simulink model "Follower_V2V_SelfSteer"  (R2014b)
settings: Solver=ode3  StartTime=0.0  StopTime=10.0  FixedStep=sampleTimes.main  RelTol=1e-3
model workspace (MAT data in the model file):
  spacing = 0
  vehicle = 0
undefined symbols (not defined in the file or in its folder): delays, sampleTimes
libraries: simulink x12
settings Model: ParameterArgumentNames=vehicle,spacing  Creator=uos  LastModifiedBy=uos

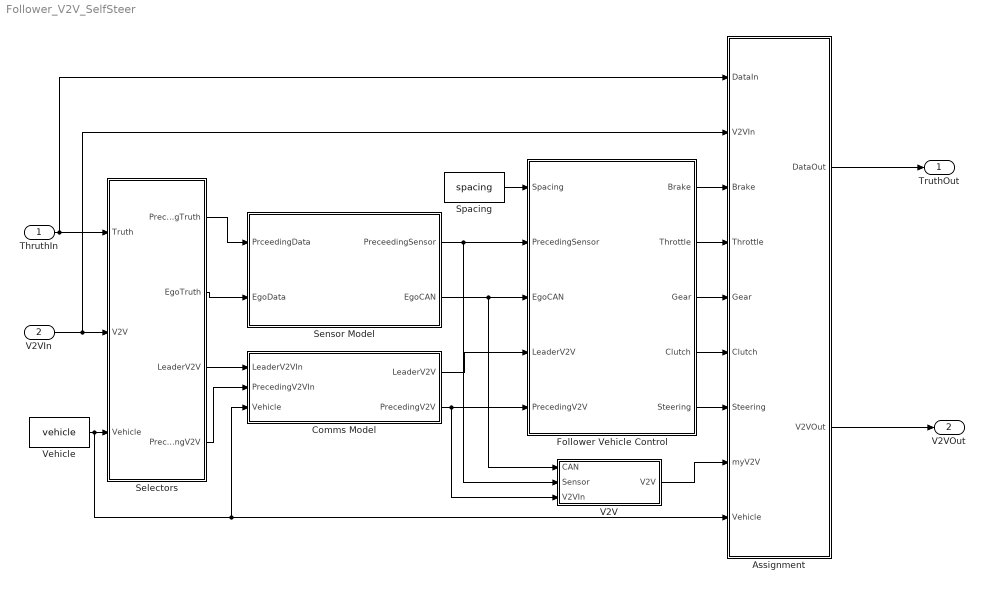
== system Follower_V2V_SelfSteer ==
  ThruthIn : Inport  OutDataTypeStr=Bus: VehicleBus  PortDimensions=10  BusOutputAsStruct=on
  V2VIn : Inport  Port=2  OutDataTypeStr=Bus: V2VBus  PortDimensions=10  SampleTime=0  BusOutputAsStruct=on
  Assignment : Subsystem
  Comms Model : Subsystem
  Follower Vehicle Control : Subsystem
  Selectors : Subsystem
  Sensor Model : Subsystem
  Spacing : Constant  Value=spacing
  V2V : Subsystem
  Vehicle : Constant  Value=vehicle
  TruthOut : Outport  OutDataTypeStr=Bus: VehicleBus  PortDimensions=10  BusOutputAsStruct=on
  V2VOut : Outport  Port=2  OutDataTypeStr=Bus: V2VBus  PortDimensions=10  BusOutputAsStruct=on
  wires:
  ThruthIn/1 -> Selectors/1(Truth), Assignment/1(DataIn)
  Assignment/1(DataOut) -> TruthOut/1
  Sensor Model/2(EgoCAN) -> V2V/1(CAN), Follower Vehicle Control/3(EgoCAN)
  Spacing/1 -> Follower Vehicle Control/1(Spacing)
  Sensor Model/1(PreceedingSensor) -> V2V/2(Sensor), Follower Vehicle Control/2(PrecedingSensor)
  Selectors/1(PrecedingTruth) -> Sensor Model/1(PrceedingData)
  Selectors/2(EgoTruth) -> Sensor Model/2(EgoData)
  Vehicle/1 -> Assignment/9(Vehicle), Comms Model/3(Vehicle), Selectors/3(Vehicle)
  Follower Vehicle Control/1(Brake) -> Assignment/3(Brake)
  Follower Vehicle Control/2(Throttle) -> Assignment/4(Throttle)
  Follower Vehicle Control/3(Gear) -> Assignment/5(Gear)
  Follower Vehicle Control/4(Clutch) -> Assignment/6(Clutch)
  Follower Vehicle Control/5(Steering) -> Assignment/7(Steering)
  Selectors/3(LeaderV2V) -> Comms Model/1(LeaderV2VIn)
  Selectors/4(PrecedingV2V) -> Comms Model/2(PrecedingV2VIn)
  Comms Model/1(LeaderV2V) -> Follower Vehicle Control/4(LeaderV2V)
  Comms Model/2(PrecedingV2V) -> V2V/3(V2VIn), Follower Vehicle Control/5(PrecedingV2V)
  V2V/1(V2V) -> Assignment/8(myV2V)
  V2VIn/1 -> Assignment/2(V2VIn), Selectors/2(V2V)
  Assignment/2(V2VOut) -> V2VOut/1

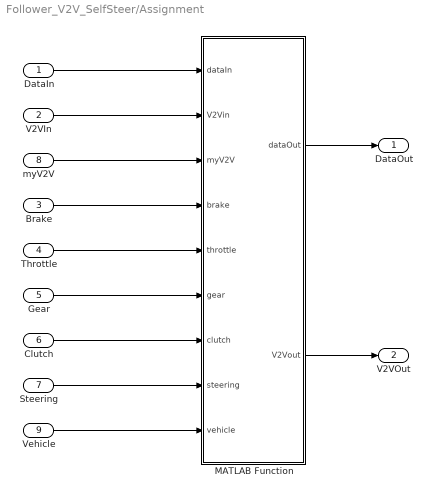
== system Follower_V2V_SelfSteer/Assignment ==
  DataIn : Inport
  V2VIn : Inport  Port=2
  Brake : Inport  Port=3
  Throttle : Inport  Port=4
  Gear : Inport  Port=5
  Clutch : Inport  Port=6
  Steering : Inport  Port=7
  myV2V : Inport  Port=8
  Vehicle : Inport  Port=9
  MATLAB Function : MATLAB Function  TreatAsAtomicUnit=on
  DataOut : Outport
  V2VOut : Outport  Port=2
  wires:
  Vehicle/1 -> MATLAB Function/9(vehicle)
  DataIn/1 -> MATLAB Function/1(dataIn)
  Brake/1 -> MATLAB Function/4(brake)
  MATLAB Function/1(dataOut) -> DataOut/1
  Throttle/1 -> MATLAB Function/5(throttle)
  Gear/1 -> MATLAB Function/6(gear)
  Clutch/1 -> MATLAB Function/7(clutch)
  Steering/1 -> MATLAB Function/8(steering)
  V2VIn/1 -> MATLAB Function/2(V2Vin)
  myV2V/1 -> MATLAB Function/3(myV2V)
  MATLAB Function/2(V2Vout) -> V2VOut/1

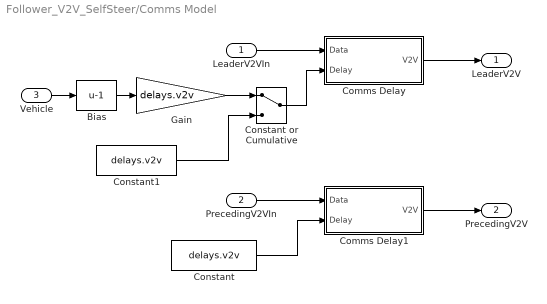
== system Follower_V2V_SelfSteer/Comms Model ==
  LeaderV2VIn : Inport
  PrecedingV2VIn : Inport  Port=2
  Vehicle : Inport  Port=3
  Bias : Bias  Bias=-1
  Comms Delay : Subsystem
  Comms Delay1 : Subsystem
  Constant : Constant  Value=delays.v2v
  Constant or Cumulative : ManualSwitch
  Constant1 : Constant  Value=delays.v2v
  Gain : Gain  Gain=delays.v2v
  LeaderV2V : Outport
  PrecedingV2V : Outport  Port=2
  wires:
  LeaderV2VIn/1 -> Comms Delay/1(Data)
  Comms Delay/1(V2V) -> LeaderV2V/1
  PrecedingV2VIn/1 -> Comms Delay1/1(Data)
  Comms Delay1/1(V2V) -> PrecedingV2V/1
  Constant/1 -> Comms Delay1/2(Delay)
  Constant or Cumulative/1 -> Comms Delay/2(Delay)
  Constant1/1 -> Constant or Cumulative/2
  Vehicle/1 -> Bias/1
  Bias/1 -> Gain/1
  Gain/1 -> Constant or Cumulative/1

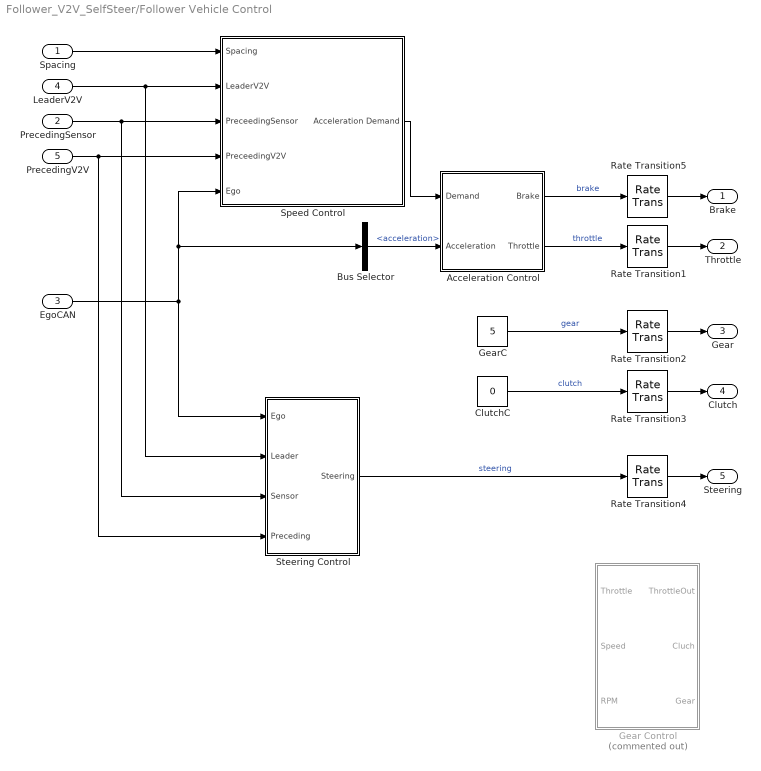
== system Follower_V2V_SelfSteer/Follower Vehicle Control ==
  Spacing : Inport
  PrecedingSensor : Inport  Port=2
  EgoCAN : Inport  Port=3
  LeaderV2V : Inport  Port=4
  PrecedingV2V : Inport  Port=5
  Acceleration Control : Subsystem
  Bus Selector : BusSelector  OutputSignals=acceleration
  ClutchC : Constant  Value=0  SampleTime=sampleTimes.control
  Gear Control : Subsystem  Commented=on
  GearC : Constant  Value=5  OutDataTypeStr=int32  SampleTime=sampleTimes.control
  Rate Transition{1..5} (5 alike) : RateTransition  OutPortSampleTime=0
  Speed Control : Subsystem
  Steering Control : Subsystem
  Brake : Outport
  Throttle : Outport  Port=2
  Gear : Outport  Port=3
  Clutch : Outport  Port=4
  Steering : Outport  Port=5
  wires:
  Acceleration Control/1(Brake) -> Rate Transition5/1  "brake"
  Bus Selector/1 -> Acceleration Control/2(Acceleration)  "<acceleration>"
  Speed Control/1(Acceleration Demand) -> Acceleration Control/1(Demand)
  Spacing/1 -> Speed Control/1(Spacing)
  EgoCAN/1 -> Speed Control/5(Ego), Bus Selector/1, Steering Control/1(Ego)
  PrecedingSensor/1 -> Steering Control/3(Sensor), Speed Control/3(PreceedingSensor)
  LeaderV2V/1 -> Steering Control/2(Leader), Speed Control/2(LeaderV2V)
  PrecedingV2V/1 -> Steering Control/4(Preceding), Speed Control/4(PreceedingV2V)
  Steering Control/1(Steering) -> Rate Transition4/1  "steering"
  Acceleration Control/2(Throttle) -> Rate Transition1/1  "throttle"
  ClutchC/1 -> Rate Transition3/1  "clutch"
  GearC/1 -> Rate Transition2/1  "gear"
  Rate Transition5/1 -> Brake/1
  Rate Transition1/1 -> Throttle/1
  Rate Transition2/1 -> Gear/1
  Rate Transition3/1 -> Clutch/1
  Rate Transition4/1 -> Steering/1

== system Follower_V2V_SelfSteer/Selectors ==
  Truth : Inport
  V2V : Inport  Port=2
  Vehicle : Inport  Port=3
  MATLAB Function : MATLAB Function  TreatAsAtomicUnit=on
  PrecedingTruth : Outport
  EgoTruth : Outport  Port=2
  LeaderV2V : Outport  Port=3
  PrecedingV2V : Outport  Port=4
  wires:
  Truth/1 -> MATLAB Function/1(data)
  Vehicle/1 -> MATLAB Function/3(vehicle)
  MATLAB Function/2(egoTruth) -> EgoTruth/1
  V2V/1 -> MATLAB Function/2(V2V)
  MATLAB Function/3(leaderV2V) -> LeaderV2V/1
  MATLAB Function/4(precedingV2V) -> PrecedingV2V/1
  MATLAB Function/1(precedingTruth) -> PrecedingTruth/1

== system Follower_V2V_SelfSteer/Sensor Model ==
  PrceedingData : Inport
  EgoData : Inport  Port=2
  CAN Model : Subsystem
  Radar Model : Subsystem
  PreceedingSensor : Outport
  EgoCAN : Outport  Port=2
  wires:
  EgoData/1 -> CAN Model/1(Data), Radar Model/2(Ego)
  PrceedingData/1 -> Radar Model/1(Target)
  Radar Model/1(Radar Data) -> PreceedingSensor/1
  CAN Model/1(CAN) -> EgoCAN/1

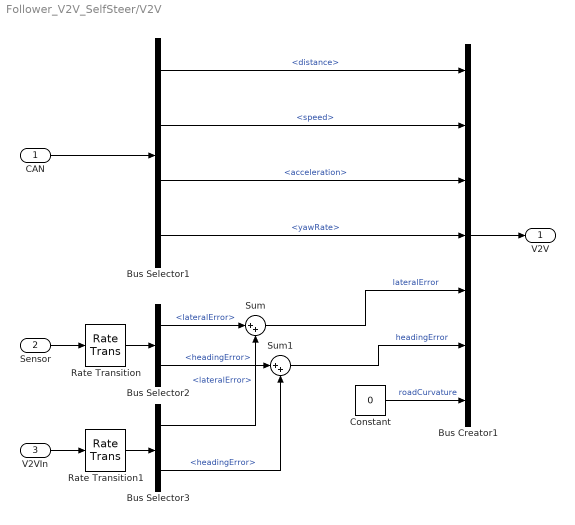
== system Follower_V2V_SelfSteer/V2V ==
  CAN : Inport
  Sensor : Inport  Port=2
  V2VIn : Inport  Port=3
  Bus Creator1 : BusCreator  Inputs=7  OutDataTypeStr=Bus: V2VBus  NonVirtualBus=on
  Bus Selector1 : BusSelector  OutputSignals=distance,speed,acceleration,yawRate
  Bus Selector2 : BusSelector  OutputSignals=lateralError,headingError
  Bus Selector3 : BusSelector  OutputSignals=lateralError,headingError
  Constant : Constant  Value=0
  Rate Transition : RateTransition  OutPortSampleTime=sampleTimes.control
  Rate Transition1 : RateTransition  OutPortSampleTime=sampleTimes.control
  Sum : Sum  Inputs=|++
  Sum1 : Sum  Inputs=|++
  V2V : Outport
  wires:
  CAN/1 -> Bus Selector1/1
  Bus Creator1/1 -> V2V/1
  Sensor/1 -> Rate Transition/1
  Bus Selector1/1 -> Bus Creator1/1  "<distance>"
  Bus Selector1/2 -> Bus Creator1/2  "<speed>"
  Bus Selector1/3 -> Bus Creator1/3  "<acceleration>"
  Bus Selector1/4 -> Bus Creator1/4  "<yawRate>"
  V2VIn/1 -> Rate Transition1/1
  Bus Selector2/1 -> Sum/1  "<lateralError>"
  Bus Selector3/1 -> Sum/2  "<lateralError>"
  Bus Selector2/2 -> Sum1/1  "<headingError>"
  Bus Selector3/2 -> Sum1/2  "<headingError>"
  Sum1/1 -> Bus Creator1/6  "headingError"
  Sum/1 -> Bus Creator1/5  "lateralError"
  Constant/1 -> Bus Creator1/7  "roadCurvature"
  Rate Transition/1 -> Bus Selector2/1
  Rate Transition1/1 -> Bus Selector3/1

== system Follower_V2V_SelfSteer/Comms Model/Comms Delay ==
  Data : Inport
  Delay : Inport  Port=2
  Rate Transition1 : RateTransition  OutPortSampleTime=sampleTimes.v2v
  Rate Transition2 : RateTransition  OutPortSampleTime=sampleTimes.main
  Variable Integer Delay : Delay  DelayLengthSource=Input port
      settings: InputPortMap=u0,p1
  Weighted Sample Time Math : SampleTimeMath  TsampMathOp=/
  V2V : Outport
  wires:
  Rate Transition1/1 -> V2V/1
  Data/1 -> Rate Transition2/1
  Rate Transition2/1 -> Variable Integer Delay/1
  Delay/1 -> Weighted Sample Time Math/1
  Weighted Sample Time Math/1 -> Variable Integer Delay/2
  Variable Integer Delay/1 -> Rate Transition1/1

== system Follower_V2V_SelfSteer/Comms Model/Comms Delay1 ==
  Data : Inport
  Delay : Inport  Port=2
  Rate Transition1 : RateTransition  OutPortSampleTime=sampleTimes.v2v
  Rate Transition2 : RateTransition  OutPortSampleTime=sampleTimes.main
  Variable Integer Delay : Delay  DelayLengthSource=Input port
      settings: InputPortMap=u0,p1
  Weighted Sample Time Math : SampleTimeMath  TsampMathOp=/
  V2V : Outport
  wires:
  Variable Integer Delay/1 -> Rate Transition1/1
  Weighted Sample Time Math/1 -> Variable Integer Delay/2
  Delay/1 -> Weighted Sample Time Math/1
  Rate Transition2/1 -> Variable Integer Delay/1
  Data/1 -> Rate Transition2/1
  Rate Transition1/1 -> V2V/1

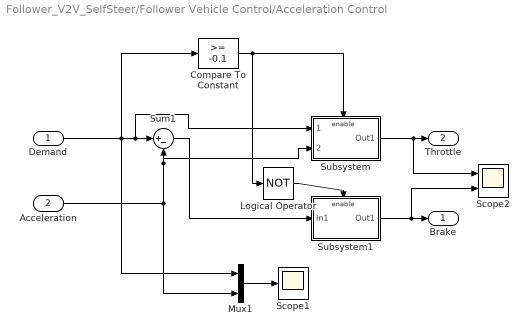
== system Follower_V2V_SelfSteer/Follower Vehicle Control/Acceleration Control ==
  Demand : Inport
  Acceleration : Inport  Port=2
  Compare To Constant : simulink/Logic and Bit Operations/Compare To Constant  relop=>=  const=-0.1  OutDataTypeStr=boolean
  Logical Operator : Logic  Operator=NOT  AllPortsSameDT=off  OutDataTypeStr=boolean
  Mux1 : Mux  Inputs=2
  Scope1 : Scope
      settings: TimeRange=3.288419527605299  YMin=-10.55000000000001  YMax=10.45000000000002  SaveName=ScopeData4
  Scope2 : Scope  NumInputPorts=2
      settings: YMin=2.5~-1  YMax=4.5~1  SaveName=ScopeData6
  Subsystem : Subsystem
  Subsystem1 : Subsystem
  Sum1 : Sum  Inputs=|+-
  Brake : Outport
  Throttle : Outport  Port=2
  wires:
  Acceleration/1 -> Subsystem/2(Acceleration), Sum1/2, Mux1/2
  Demand/1 -> Compare To Constant/1, Mux1/1, Subsystem/1(Demand), Sum1/1
  Sum1/1 -> Subsystem1/1(In1)
  Subsystem1/1(Out1) -> Scope2/2, Brake/1
  Mux1/1 -> Scope1/1
  Subsystem/1(Out1) -> Scope2/1, Throttle/1
  Compare To Constant/1 -> Subsystem/Enable, Logical Operator/1
  Logical Operator/1 -> Subsystem1/Enable

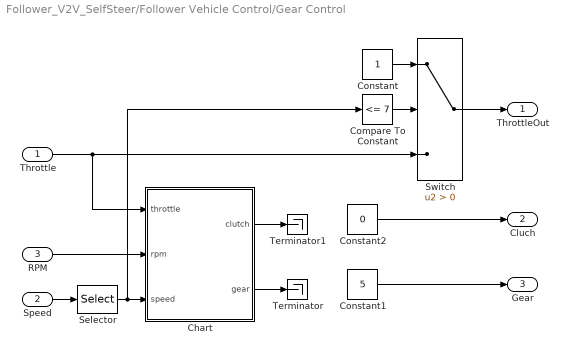
== system Follower_V2V_SelfSteer/Follower Vehicle Control/Gear Control ==
  Throttle : Inport
  Speed : Inport  Port=2
  RPM : Inport  Port=3
  Chart : Stateflow chart  TreatAsAtomicUnit=on
  Compare To Constant : simulink/Logic and Bit Operations/Compare To Constant  relop=<=  const=7  OutDataTypeStr=boolean
  Constant : Constant  OutDataTypeStr=single
  Constant1 : Constant  Value=5  OutDataTypeStr=int32
  Constant2 : Constant  Value=0  OutDataTypeStr=double
  Selector : Selector  InputPortWidth=3
  Switch : Switch  Criteria=u2 > Threshold
  Terminator : Terminator
  Terminator1 : Terminator
  ThrottleOut : Outport
  Cluch : Outport  Port=2
  Gear : Outport  Port=3
  wires:
  Constant2/1 -> Cluch/1
  Constant1/1 -> Gear/1
  Switch/1 -> ThrottleOut/1
  Constant/1 -> Switch/1
  RPM/1 -> Chart/2(rpm)
  Throttle/1 -> Chart/1(throttle), Switch/3
  Speed/1 -> Selector/1
  Selector/1 -> Chart/3(speed), Compare To Constant/1
  Compare To Constant/1 -> Switch/2
  Chart/2(gear) -> Terminator/1
  Chart/1(clutch) -> Terminator1/1

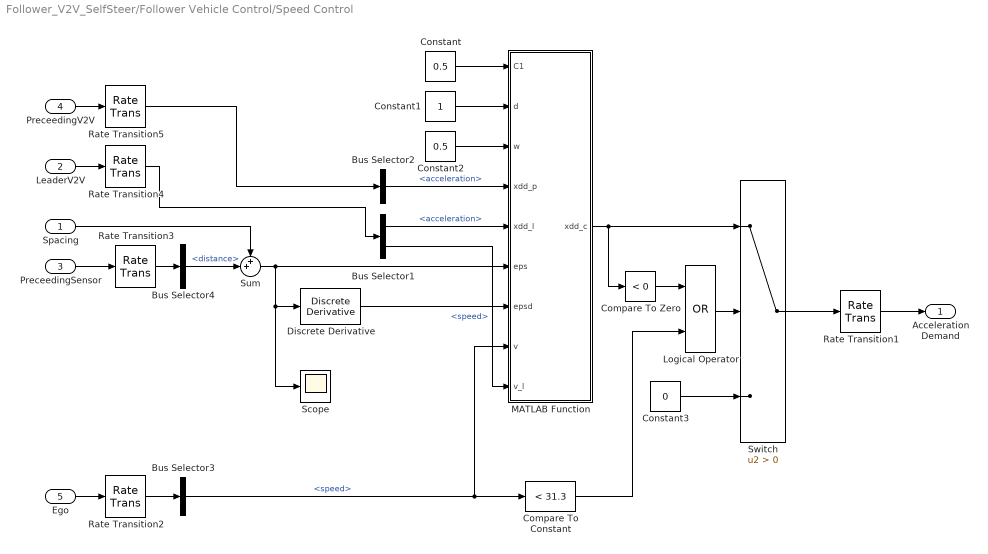
== system Follower_V2V_SelfSteer/Follower Vehicle Control/Speed Control ==
  Spacing : Inport
  LeaderV2V : Inport  Port=2
  PreceedingSensor : Inport  Port=3
  PreceedingV2V : Inport  Port=4
  Ego : Inport  Port=5
  Bus Selector1 : BusSelector  OutputSignals=acceleration,speed
  Bus Selector2 : BusSelector  OutputSignals=acceleration
  Bus Selector3 : BusSelector  OutputSignals=speed
  Bus Selector4 : BusSelector  OutputSignals=distance
  Compare To Constant : simulink/Logic and Bit Operations/Compare To Constant  relop=<  const=31.3  OutDataTypeStr=boolean
  Compare To Zero : simulink/Logic and Bit Operations/Compare To Zero  relop=<  OutDataTypeStr=boolean
  Constant : Constant  Value=0.5
  Constant1 : Constant
  Constant2 : Constant  Value=0.5
  Constant3 : Constant  Value=0
  Discrete Derivative : simulink/Discrete/Discrete Derivative  gainval=1.0  ICPrevScaledInput=0.0  InputProcessing=Inherited  OutMin=[]  OutMax=[]  OutDataType=fixdt(1, 16)  OutScaling=2^-10  DoSatur=off
  Logical Operator : Logic  Operator=OR  AllPortsSameDT=off  OutDataTypeStr=boolean
  MATLAB Function : MATLAB Function  TreatAsAtomicUnit=on
  Rate Transition1 : RateTransition  Deterministic=off
  Rate Transition{2..5} (4 alike) : RateTransition  OutPortSampleTime=sampleTimes.control
  Scope : Scope
      settings: TimeRange=10  YMin=-0.05  YMax=0.2
  Sum : Sum  Inputs=++|
  Switch : Switch  Criteria=u2 > Threshold
  Acceleration Demand : Outport
  wires:
  Compare To Zero/1 -> Logical Operator/1
  Logical Operator/1 -> Switch/2
  Ego/1 -> Rate Transition2/1
  Bus Selector3/1 -> Compare To Constant/1, MATLAB Function/8(v)  "<speed>"
  Compare To Constant/1 -> Logical Operator/2
  Constant3/1 -> Switch/3
  PreceedingSensor/1 -> Rate Transition3/1
  Bus Selector4/1 -> Sum/2  "<distance>"
  Sum/1 -> MATLAB Function/6(eps), Scope/1, Discrete Derivative/1
  MATLAB Function/1(xdd_c) -> Switch/1, Compare To Zero/1
  Switch/1 -> Rate Transition1/1
  Discrete Derivative/1 -> MATLAB Function/7(epsd)
  Rate Transition1/1 -> Acceleration Demand/1
  Constant/1 -> MATLAB Function/1(C1)
  Constant1/1 -> MATLAB Function/2(d)
  Constant2/1 -> MATLAB Function/3(w)
  Spacing/1 -> Sum/1
  LeaderV2V/1 -> Rate Transition4/1
  Bus Selector1/1 -> MATLAB Function/5(xdd_l)  "<acceleration>"
  Bus Selector1/2 -> MATLAB Function/9(v_l)  "<speed>"
  PreceedingV2V/1 -> Rate Transition5/1
  Bus Selector2/1 -> MATLAB Function/4(xdd_p)  "<acceleration>"
  Rate Transition2/1 -> Bus Selector3/1
  Rate Transition3/1 -> Bus Selector4/1
  Rate Transition4/1 -> Bus Selector1/1
  Rate Transition5/1 -> Bus Selector2/1

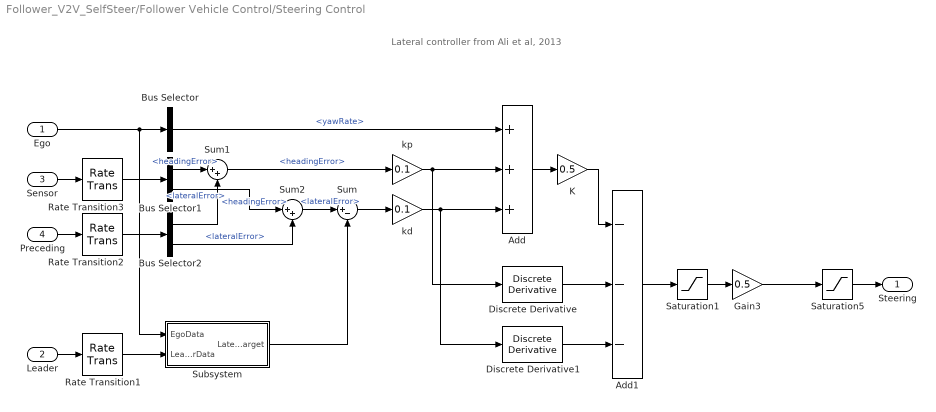
== system Follower_V2V_SelfSteer/Follower Vehicle Control/Steering Control ==
  note: Lateral controller from Ali et al, 2013
  Ego : Inport
  Leader : Inport  Port=2
  Sensor : Inport  Port=3
  Preceding : Inport  Port=4
  Add : Sum  Inputs=+++
  Add1 : Sum  Inputs=---
  Bus Selector : BusSelector  OutputSignals=yawRate
  Bus Selector1 : BusSelector  OutputSignals=headingError,lateralError
  Bus Selector2 : BusSelector  OutputSignals=headingError,lateralError
  Discrete Derivative : simulink/Discrete/Discrete Derivative  gainval=1.0  ICPrevScaledInput=0.0  InputProcessing=Inherited  OutMin=[]  OutMax=[]  OutDataType=fixdt(1, 16)  OutScaling=2^-10  DoSatur=off
  Discrete Derivative1 : simulink/Discrete/Discrete Derivative  gainval=1.0  ICPrevScaledInput=0.0  InputProcessing=Inherited  OutMin=[]  OutMax=[]  OutDataType=fixdt(1, 16)  OutScaling=2^-10  DoSatur=off
  Gain3 : Gain  Gain=0.5
  K : Gain  Gain=0.5
  Rate Transition1 : RateTransition  OutPortSampleTime=sampleTimes.control
  Rate Transition2 : RateTransition  OutPortSampleTime=sampleTimes.control
  Rate Transition3 : RateTransition  OutPortSampleTime=sampleTimes.control
  Saturation1 : Saturate  UpperLimit=0.02  LowerLimit=-0.02
  Saturation5 : Saturate
  Subsystem : Subsystem
  Sum : Sum  Inputs=|+-
  Sum1 : Sum  Inputs=|++
  Sum2 : Sum  Inputs=|++
  kd : Gain  Gain=0.1
  kp : Gain  Gain=0.1
  Steering : Outport
  wires:
  Ego/1 -> Subsystem/1(EgoData), Bus Selector/1
  Leader/1 -> Rate Transition1/1
  Saturation1/1 -> Gain3/1
  Sum/1 -> kd/1
  Add1/1 -> Saturation1/1
  K/1 -> Add1/1
  Discrete Derivative1/1 -> Add1/3
  Discrete Derivative/1 -> Add1/2
  Add/1 -> K/1
  kp/1 -> Add/2, Discrete Derivative/1
  kd/1 -> Add/3, Discrete Derivative1/1
  Sum2/1 -> Sum/1  "<lateralError>"
  Sum1/1 -> kp/1  "<headingError>"
  Gain3/1 -> Saturation5/1
  Saturation5/1 -> Steering/1
  Bus Selector/1 -> Add/1  "<yawRate>"
  Subsystem/1(Lateral Target) -> Sum/2
  Sensor/1 -> Rate Transition3/1
  Preceding/1 -> Rate Transition2/1
  Bus Selector1/1 -> Sum1/1  "<headingError>"
  Bus Selector2/1 -> Sum1/2  "<headingError>"
  Bus Selector1/2 -> Sum2/1  "<lateralError>"
  Bus Selector2/2 -> Sum2/2  "<lateralError>"
  Rate Transition1/1 -> Subsystem/2(LeaderData)
  Rate Transition2/1 -> Bus Selector2/1
  Rate Transition3/1 -> Bus Selector1/1

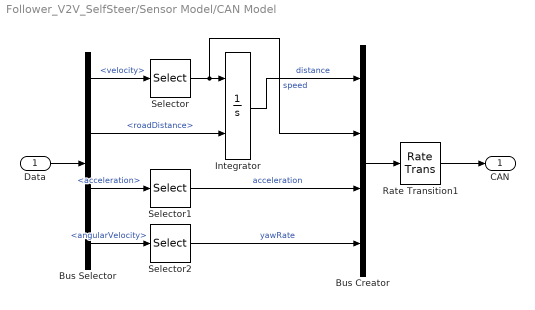
== system Follower_V2V_SelfSteer/Sensor Model/CAN Model ==
  Data : Inport
  Bus Creator : BusCreator
  Bus Selector : BusSelector  OutputSignals=data.velocity,data.roadDistance,data.acceleration,data.angularVelocity
  Integrator : Integrator  InitialConditionSource=external
  Rate Transition1 : RateTransition  OutPortSampleTime=sampleTimes.main
  Selector : Selector  InputPortWidth=3
  Selector1 : Selector  InputPortWidth=3
  Selector2 : Selector  InputPortWidth=3
  CAN : Outport
  wires:
  Rate Transition1/1 -> CAN/1
  Bus Creator/1 -> Rate Transition1/1
  Selector1/1 -> Bus Creator/3  "acceleration"
  Bus Selector/3 -> Selector1/1  "<acceleration>"
  Integrator/1 -> Bus Creator/1  "distance"
  Selector/1 -> Integrator/1, Bus Creator/2  "speed"
  Bus Selector/1 -> Selector/1  "<velocity>"
  Data/1 -> Bus Selector/1
  Bus Selector/2 -> Integrator/2  "<roadDistance>"
  Bus Selector/4 -> Selector2/1  "<angularVelocity>"
  Selector2/1 -> Bus Creator/4  "yawRate"

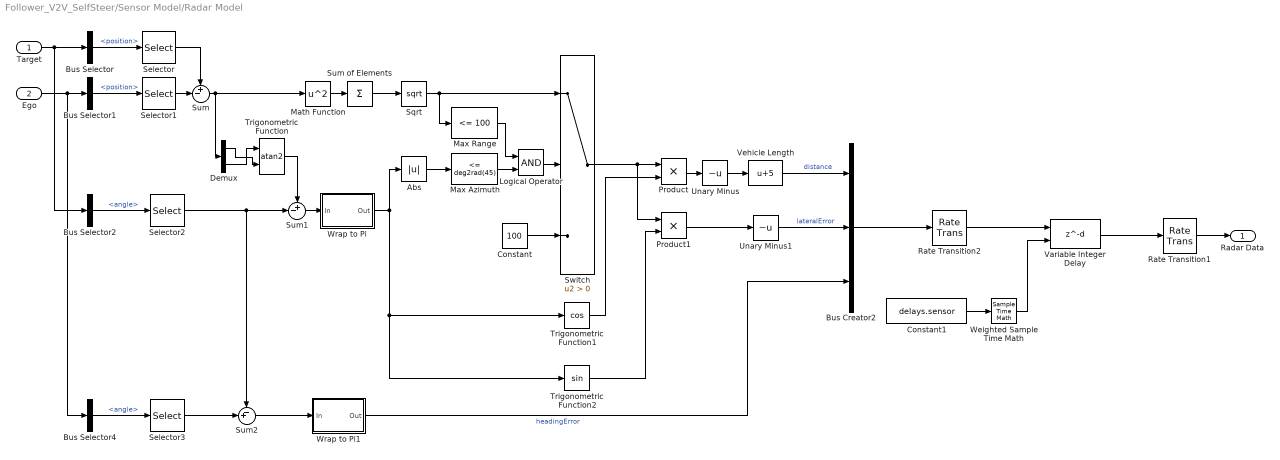
== system Follower_V2V_SelfSteer/Sensor Model/Radar Model ==
  Target : Inport
  Ego : Inport  Port=2
  Abs : Abs
  Bus Creator2 : BusCreator  Inputs=3
  Bus Selector : BusSelector  OutputSignals=data.position
  Bus Selector1 : BusSelector  OutputSignals=data.position
  Bus Selector2 : BusSelector  OutputSignals=data.angle
  Bus Selector4 : BusSelector  OutputSignals=data.angle
  Constant : Constant  Value=100
  Constant1 : Constant  Value=delays.sensor
  Demux : Demux  Outputs=2
  Logical Operator : Logic  AllPortsSameDT=off  OutDataTypeStr=boolean
  Math Function : Math  Operator=square  SaturateOnIntegerOverflow=on
  Max Azimuth : simulink/Logic and Bit Operations/Compare To Constant  relop=<=  const=deg2rad(45)  OutDataTypeStr=boolean
  Max Range : simulink/Logic and Bit Operations/Compare To Constant  relop=<=  const=100  OutDataTypeStr=boolean
  Product : Product
  Product1 : Product
  Rate Transition1 : RateTransition  OutPortSampleTime=sampleTimes.sensor
  Rate Transition2 : RateTransition  OutPortSampleTime=sampleTimes.main
  Selector : Selector  InputPortWidth=3  Indices=[1 2]
  Selector1 : Selector  InputPortWidth=3  Indices=[1 2]
  Selector2 : Selector  InputPortWidth=3  Indices=3
  Selector3 : Selector  InputPortWidth=3  Indices=3
  Sqrt : Sqrt  SaturateOnIntegerOverflow=on
  Sum : Sum  Inputs=+-|
  Sum of Elements : Sum  Inputs=+
  Sum1 : Sum  Inputs=+-|
  Sum2 : Sum  Inputs=-+|
  Switch : Switch  Criteria=u2 > Threshold
  Trigonometric Function : Trigonometry  Operator=atan2
  Trigonometric Function1 : Trigonometry  Operator=cos
  Trigonometric Function2 : Trigonometry
  Unary Minus : UnaryMinus
  Unary Minus1 : UnaryMinus
  Variable Integer Delay : Delay  DelayLengthSource=Input port
      settings: InputPortMap=u0,p1
  Vehicle Length : Bias  Bias=5
  Weighted Sample Time Math : SampleTimeMath  TsampMathOp=/
  Wrap to Pi : Subsystem
  Wrap to Pi1 : Subsystem
  Radar Data : Outport
  wires:
  Selector1/1 -> Sum/2
  Selector/1 -> Sum/1
  Target/1 -> Bus Selector2/1, Bus Selector/1
  Bus Selector/1 -> Selector/1  "<position>"
  Bus Selector1/1 -> Selector1/1  "<position>"
  Ego/1 -> Bus Selector4/1, Bus Selector1/1
  Bus Selector2/1 -> Selector2/1  "<angle>"
  Sum/1 -> Math Function/1, Demux/1
  Selector2/1 -> Sum2/1, Sum1/2
  Trigonometric Function/1 -> Sum1/1
  Sum1/1 -> Wrap to Pi/1(In)
  Math Function/1 -> Sum of Elements/1
  Sum of Elements/1 -> Sqrt/1
  Constant/1 -> Switch/3
  Sqrt/1 -> Max Range/1, Switch/1
  Logical Operator/1 -> Switch/2
  Max Range/1 -> Logical Operator/1
  Abs/1 -> Max Azimuth/1
  Max Azimuth/1 -> Logical Operator/2
  Switch/1 -> Product1/1, Product/1
  Trigonometric Function1/1 -> Product/2
  Trigonometric Function2/1 -> Product1/2
  Product/1 -> Unary Minus/1
  Demux/1 -> Trigonometric Function/2
  Demux/2 -> Trigonometric Function/1
  Wrap to Pi/1(Out) -> Trigonometric Function2/1, Trigonometric Function1/1, Abs/1
  Unary Minus/1 -> Vehicle Length/1
  Bus Creator2/1 -> Rate Transition2/1
  Rate Transition1/1 -> Radar Data/1
  Vehicle Length/1 -> Bus Creator2/1  "distance"
  Product1/1 -> Unary Minus1/1
  Rate Transition2/1 -> Variable Integer Delay/1
  Variable Integer Delay/1 -> Rate Transition1/1
  Constant1/1 -> Weighted Sample Time Math/1
  Weighted Sample Time Math/1 -> Variable Integer Delay/2
  Bus Selector4/1 -> Selector3/1  "<angle>"
  Selector3/1 -> Sum2/2
  Sum2/1 -> Wrap to Pi1/1(In)
  Unary Minus1/1 -> Bus Creator2/2  "lateralError"
  Wrap to Pi1/1(Out) -> Bus Creator2/3  "headingError"

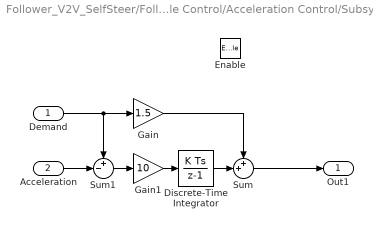
== system Follower_V2V_SelfSteer/Follower Vehicle Control/Acceleration Control/Subsystem ==
  Demand : Inport
  Acceleration : Inport  Port=2
  Enable : EnablePort  StatesWhenEnabling=reset
  Discrete-Time Integrator : DiscreteIntegrator  InitialConditionSetting=State (most efficient)  SampleTime=-1  LimitOutput=on  UpperSaturationLimit=1  LowerSaturationLimit=-1
  Gain : Gain  Gain=1.5
  Gain1 : Gain  Gain=10
  Sum : Sum  Inputs=++|
  Sum1 : Sum  Inputs=+-|
  Out1 : Outport  OutputWhenDisabled=reset  InitialOutput=0
  wires:
  Gain/1 -> Sum/1
  Discrete-Time Integrator/1 -> Sum/2
  Gain1/1 -> Discrete-Time Integrator/1
  Sum/1 -> Out1/1
  Demand/1 -> Sum1/1, Gain/1
  Acceleration/1 -> Sum1/2
  Sum1/1 -> Gain1/1

== system Follower_V2V_SelfSteer/Follower Vehicle Control/Acceleration Control/Subsystem1 ==
  In1 : Inport
  Enable : EnablePort  StatesWhenEnabling=reset
  Discrete-Time Integrator : DiscreteIntegrator  InitialConditionSetting=State (most efficient)  SampleTime=-1  LimitOutput=on  UpperSaturationLimit=1  LowerSaturationLimit=-1
  Gain2 : Gain  Gain=0.005
  Gain3 : Gain
  Saturation1 : Saturate  UpperLimit=1  LowerLimit=0
  Sum2 : Sum  Inputs=++|
  Unary Minus : UnaryMinus
  Out1 : Outport  OutputWhenDisabled=reset  InitialOutput=0
  wires:
  Saturation1/1 -> Out1/1
  Sum2/1 -> Saturation1/1
  In1/1 -> Unary Minus/1
  Gain2/1 -> Sum2/2
  Discrete-Time Integrator/1 -> Sum2/1
  Gain3/1 -> Discrete-Time Integrator/1
  Unary Minus/1 -> Gain2/1, Gain3/1

== system Follower_V2V_SelfSteer/Follower Vehicle Control/Steering Control/Subsystem ==
  EgoData : Inport
  LeaderData : Inport  Port=2
  Bus Selector : BusSelector  OutputSignals=distance
  Bus Selector1 : BusSelector  OutputSignals=distance,lateralError
  Lookup Table Dynamic : simulink/Lookup Tables/Lookup Table Dynamic  Commented=on  LookUpMeth=Interpolation-Use End Values  OutDataTypeStr=fixdt('double')  OutputDataTypeScalingMode=Specify via dialog  OutDataType=fixdt('double')  OutScaling=2^-10  DoSatur=off
  Tapped Delay : simulink/Discrete/Tapped Delay  vinit=0.0  samptime=-1  NumDelays=1000  DelayOrder=Oldest  includeCurrent=off
  Tapped Delay1 : simulink/Discrete/Tapped Delay  vinit=0.0  samptime=-1  NumDelays=1000  DelayOrder=Oldest  includeCurrent=off
  Lateral Target : Outport
  wires:
  Bus Selector1/1 -> Tapped Delay1/1  "<distance>"
  Bus Selector1/2 -> Lateral Target/1, Tapped Delay/1  "<lateralError>"
  EgoData/1 -> Bus Selector/1
  LeaderData/1 -> Bus Selector1/1
  Bus Selector/1 -> Lookup Table Dynamic/1  "<distance>"
  Tapped Delay1/1 -> Lookup Table Dynamic/2
  Tapped Delay/1 -> Lookup Table Dynamic/3

== system Follower_V2V_SelfSteer/Sensor Model/Radar Model/Wrap to Pi ==
  In : Inport
  Bias : Bias  Bias=pi
  Bias1 : Bias  Bias=-pi
  Constant : Constant  Value=2*pi
  Math Function : Math  Operator=mod  SaturateOnIntegerOverflow=on
  Out : Outport
  wires:
  In/1 -> Bias/1
  Bias/1 -> Math Function/1
  Math Function/1 -> Bias1/1
  Bias1/1 -> Out/1
  Constant/1 -> Math Function/2

== system Follower_V2V_SelfSteer/Sensor Model/Radar Model/Wrap to Pi1 ==
  In : Inport
  Bias : Bias  Bias=pi
  Bias1 : Bias  Bias=-pi
  Constant : Constant  Value=2*pi
  Math Function : Math  Operator=mod  SaturateOnIntegerOverflow=on
  Out : Outport
  wires:
  Constant/1 -> Math Function/2
  Bias1/1 -> Out/1
  Math Function/1 -> Bias1/1
  Bias/1 -> Math Function/1
  In/1 -> Bias/1

== matlab function Follower_V2V_SelfSteer/Assignment/MATLAB Function ==
  data: dataIn input Bus: VehicleBus size=10; V2Vin input Bus: V2VBus size=10; myV2V input Bus: V2VBus size=1; brake input size=1; throttle input; gear input; clutch input; steering input; dataOut output Bus: VehicleBus size=10; vehicle input; V2Vout output Bus: V2VBus size=10
function [dataOut, V2Vout]  = fcn(dataIn, V2Vin, myV2V, brake,throttle,gear,clutch,steering, vehicle)
%#codegen

dataOut = dataIn;
dataOut(vehicle).control.brake = brake;
dataOut(vehicle).control.throttle = throttle;
dataOut(vehicle).control.clutch = clutch;
dataOut(vehicle).control.steering = steering;
dataOut(vehicle).control.gear = gear;

V2Vout = V2Vin;
V2Vout(vehicle) = myV2V;

== matlab function Follower_V2V_SelfSteer/Selectors/MATLAB Function ==
  data: precedingTruth output Bus: VehicleBus size=1; egoTruth output Bus: VehicleBus size=1; leaderV2V output Bus: V2VBus size=1; data input Bus: VehicleBus size=10; V2V input Bus: V2VBus size=10; precedingV2V output Bus: V2VBus size=1; vehicle input
function [precedingTruth, egoTruth, leaderV2V, precedingV2V] = fcn(data, V2V, vehicle)
%#codegen

if (vehicle > 1)
    precedingTruth = data(vehicle-1);
    precedingV2V = V2V(vehicle-1);
else
    error('There is no preceeding vehicle!');
end
egoTruth = data(vehicle);

leaderV2V = V2V(1);

== stateflow chart Follower_V2V_SelfSteer/Follower Vehicle Control/Gear Control/Chart ==
  state ShiftLogic [parallel]
    en: gear = int32(1); minRPM = 2000; maxRPM = 6000;
    settings: executionOrder=1
    state Downshift
      en:clutch = 1;
      ex: gear = gear - int32(1);
    state SteadyState
      en: clutch =0;
    state Upshift
      en: clutch = 1;
      ex: gear = gear + int32(1);
    state Cruise
      en: clutch = 1;
      ex: gear = int32(5);
    (default) -> SteadyState
    SteadyState -> Upshift [order 2] : after(100,msec)[gear < 5 && (rpm > maxRPM || (throttle < 0.25 && rpm > minRPM))]
    SteadyState -> Downshift [order 3] : after(100,msec)[speed < 15 && throttle > 0.25 && (gear > 1 && rpm < minRPM)]
    Upshift -> SteadyState : after(100,msec)
    Downshift -> SteadyState : after(100,msec)
    Cruise -> SteadyState : after(100,msec)
    SteadyState -> Cruise [order 1] : [gear ~=5 && speed > 15]
  data: throttle input; rpm input; clutch output double; minRPM local; maxRPM local; gear output int32; speed input

== matlab function Follower_V2V_SelfSteer/Follower Vehicle Control/Speed Control/MATLAB Function ==
  data: C1 input; d input; w input; xdd_p input; xdd_c output; xdd_l input; eps input; epsd input; v input; v_l input
function xdd_c = fcn(C1, d, w, xdd_p, xdd_l, eps, epsd, v, v_l)
%#codegen

xdd_c = (1-C1)*xdd_p + C1*xdd_l - (2*d - C1*(d + sqrt(d*d - 1)))*w*epsd ...
    - (d + sqrt(d*d - 1))*w*C1*(v-v_l) - w*w*eps;
